simulink model "gctest"  (Simulink 6.2)
settings: Solver=ode45  StartTime=0.0  StopTime=10  RelTol=1e-3
libraries: components_lib x5, simulink x1
settings Model: LastModifiedBy=Mads
settings DebuggingCC: SolverPrmCheckMsg=warning

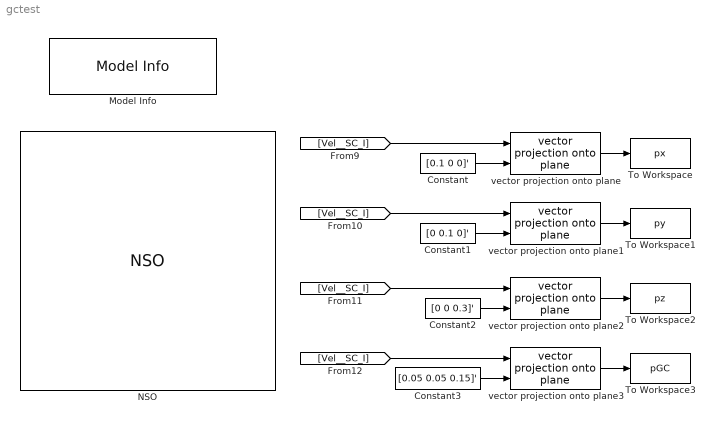
== system gctest ==
  Constant : Constant  Value=[0.1 0 0]'
  Constant1 : Constant  Value=[0 0.1 0]'
  Constant2 : Constant  Value=[0 0 0.3]'
  Constant3 : Constant  Value=[0.05 0.05 0.15]'
  Model Info : simulink/Model-Wide Utilities/Model Info  InitialBlockCM=None  BlockCM=None  Frame=on  DisplayStringWithTags=|  HorizontalTextAlignment=Center  LeftAlignmentValue=0.5  SourceBlockDiagram=gctest  TagMaxNumber=20
      | sun to eclipse : 2452315.560376
      | 32 sec. before : 2452315.56
      | eclipse to sun : 2452315.513363
  NSO : components_lib/NSO  Tag=AAUSAT-II Model  Description=AAUSAT-II Model  r_com_s=[0.05 0.05 0.15]  sat_temp_start=0  r_com_s_deployed=[0.05 0.05 0.125]  mass_sc=3  Dim=[0.1 0.1 0.3]  inertia_c=[25 25 5]/1e3  inertia_d=[42.3 42.3 28.4]/1e3  init_jd=2452315.56  q_s_c=[0 0 0 1]  q_init_s_i=[sqrt(0.5) 0 0 sqrt(0.5)]  w_init_s=[0.1 0.1 0.1]*0  Cd=2  rho=9.25e-13  enable_sensor_emulation=off  alb_emu_enabled=off  enable_dist=off
  To Workspace : ToWorkspace  VariableName=px  SampleTime=-1  SaveFormat=Structure
  To Workspace1 : ToWorkspace  VariableName=py  SampleTime=-1  SaveFormat=Structure
  To Workspace2 : ToWorkspace  VariableName=pz  SampleTime=-1  SaveFormat=Structure
  To Workspace3 : ToWorkspace  VariableName=pGC  SampleTime=-1  SaveFormat=Structure
  vector projection onto plane{,1..3} (4 alike) : components_lib/Math utilities/Vector operations/vector projection onto plane
  wires:
  [Vel__SC_I] -> vector projection onto plane1/1
  [Vel__SC_I] -> vector projection onto plane2/1
  [Vel__SC_I] -> vector projection onto plane/1
  vector projection onto plane2/1 -> To Workspace2/1
  vector projection onto plane1/1 -> To Workspace1/1
  Constant2/1 -> vector projection onto plane2/2
  Constant1/1 -> vector projection onto plane1/2
  Constant/1 -> vector projection onto plane/2
  vector projection onto plane/1 -> To Workspace/1
  [Vel__SC_I] -> vector projection onto plane3/1
  vector projection onto plane3/1 -> To Workspace3/1
  Constant3/1 -> vector projection onto plane3/2
